simulink model "MiniDroneLogicalArchitecture_Initial"  (R2022a)
settings: Solver=VariableStepAuto  StartTime=0.0  StopTime=10.0  RelTol=1e-3
settings Model: DataDictionary=MiniDroneArchData.sldd  Creator=tshifera  LastModifiedBy=31630

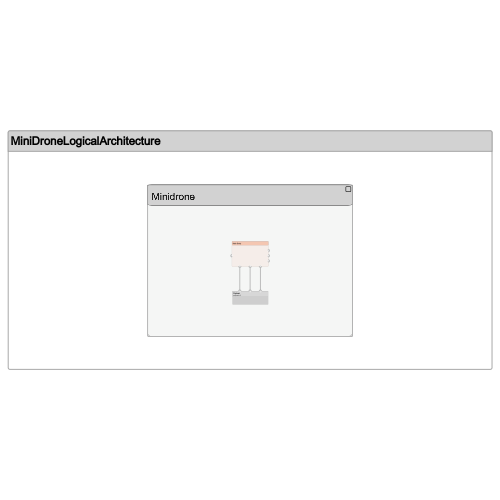
[thumbnail: Simulink's stored preview of the top-level diagram]
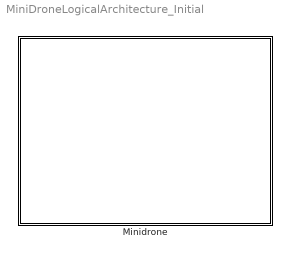
== system MiniDroneLogicalArchitecture_Initial ==
  Minidrone : Subsystem
      settings: PortSchema="{\"entries\":[{\"content\":{\"headerSize\":26,\"margin\":15,\"minimumSpacing\":25,\"sides\":[{\"content\":{\"connectorIds\":[]},\"type\":\"ConnectorPlacement.EquallySpacedRectSide\",\"uuid\":\"58971a95-43ec-4e42-90cb-f52848a43a78\"},{\"content\":{\"connectorIds\":[],\"side\":\"RIGHT\"},\"type\":\"ConnectorPlacement.EquallySpacedRectSide\",\"uuid\":\"43bd139b-3ebd-443e-9d04-2758c166e5e5\"},{\"content\":{\"connectorIds\":[],\"side\":\"TOP\"},\"type\":\"ConnectorPlacement.EquallySpacedRectSide\",\"uuid\":\"9440dd5a-d47a-4e7e-9dec-7137884490cd\"}]},\"type\":\"ConnectorPlacement.EquallySpacedConnector\",\"uuid\":\"fbcd83c6-9a27-4688-9f1d-1a4d28d86620\"}],\"packageUris\":[\"http://schema.mathworks.com/mf0/Connector/R2020b\"],\"version\":\"1.0\"}"

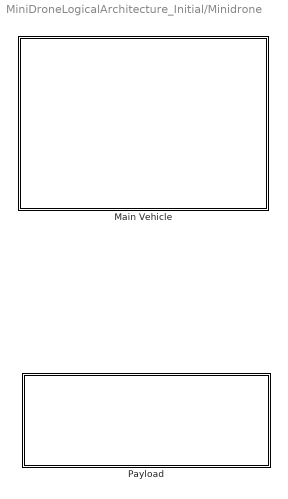
== system MiniDroneLogicalArchitecture_Initial/Minidrone ==
  Main Vehicle : Subsystem
      settings: PortSchema="{\"entries\":[{\"content\":{\"headerSize\":26,\"margin\":15,\"minimumSpacing\":25,\"sides\":[{\"content\":{\"connectorIds\":[]},\"type\":\"ConnectorPlacement.EquallySpacedRectSide\",\"uuid\":\"58971a95-43ec-4e42-90cb-f52848a43a78\"},{\"content\":{\"connectorIds\":[],\"side\":\"RIGHT\"},\"type\":\"ConnectorPlacement.EquallySpacedRectSide\",\"uuid\":\"43bd139b-3ebd-443e-9d04-2758c166e5e5\"},{\"content\":{\"connectorIds\":[],\"side\":\"TOP\"},\"type\":\"ConnectorPlacement.EquallySpacedRectSide\",\"uuid\":\"9440dd5a-d47a-4e7e-9dec-7137884490cd\"},{\"content\":{\"connectorIds\":[],\"side\":\"BOTTOM\"},\"type\":\"ConnectorPlacement.EquallySpacedRectSide\",\"uuid\":\"027f250f-1c99-4780-b31a-0472dacd58c4\"}]},\"type\":\"ConnectorPlacement.EquallySpacedConnector\",\"uuid\":\"fbcd83c6-9a27-4688-9f1d-1a4d28d86620\"}],\"packageUris\":[\"http://schema.mathworks.com/mf0/Connector/R2020b\"],\"version\":\"1.0\"}"
  Payload : Subsystem  Variant=on
      settings: PortSchema="{\"entries\":[{\"content\":{\"headerSize\":38,\"margin\":15,\"minimumSpacing\":25,\"sides\":[{\"content\":{\"connectorIds\":[]},\"type\":\"ConnectorPlacement.EquallySpacedRectSide\",\"uuid\":\"bb20ca61-cc69-46ba-bbf8-c616735728e4\"},{\"content\":{\"connectorIds\":[],\"side\":\"RIGHT\"},\"type\":\"ConnectorPlacement.EquallySpacedRectSide\",\"uuid\":\"ae599026-5f79-458c-a34f-615f09cd605e\"},{\"content\":{\"connectorIds\":[],\"side\":\"TOP\"},\"type\":\"ConnectorPlacement.EquallySpacedRectSide\",\"uuid\":\"37784589-cb93-414b-b17d-4791bb265658\"}]},\"type\":\"ConnectorPlacement.EquallySpacedConnector\",\"uuid\":\"a9e16083-13fe-49b9-9fa3-3eed0fc58f12\"}],\"packageUris\":[\"http://schema.mathworks.com/mf0/Connector/R2020b\"],\"version\":\"1.0\"}"

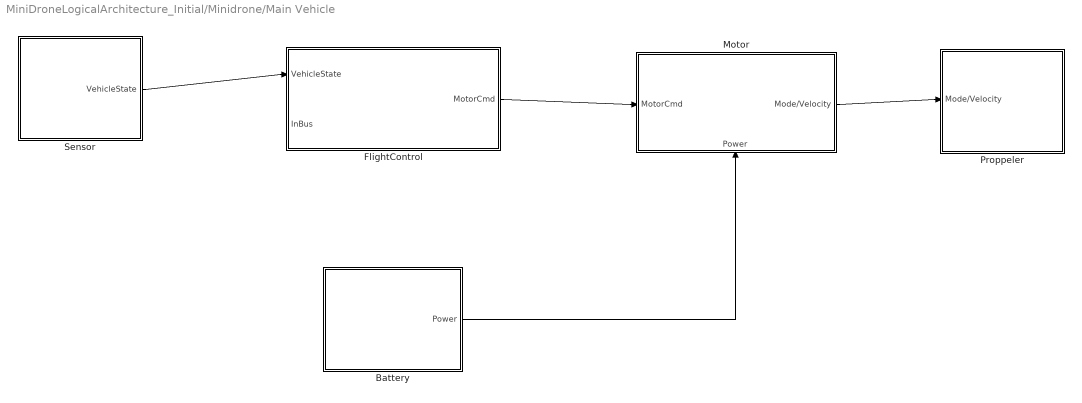
== system MiniDroneLogicalArchitecture_Initial/Minidrone/Main Vehicle ==
  Battery : Subsystem
      settings: PortSchema="{\"entries\":[{\"content\":{\"headerSize\":26,\"margin\":15,\"minimumSpacing\":25,\"sides\":[{\"content\":{\"connectorIds\":[]},\"type\":\"ConnectorPlacement.EquallySpacedRectSide\",\"uuid\":\"0bc5e52b-da78-4400-aa5e-9dddd6e99de1\"},{\"content\":{\"connectorIds\":[\"Out1\"],\"side\":\"RIGHT\"},\"type\":\"ConnectorPlacement.EquallySpacedRectSide\",\"uuid\":\"07f8a464-8fcf-4142-a2f1-5b89308ee41c\"},{\"content\":{\"connectorIds\":[],\"side\":\"TOP\"},\"type\":\"ConnectorPlacement.EquallySpacedRectSide\",\"uuid\":\"c21b697f-1019-46e9-b9d1-38a67279521c\"}]},\"type\":\"ConnectorPlacement.EquallySpacedConnector\",\"uuid\":\"700f190d-f37a-482f-bf2b-8de029522908\"}],\"packageUris\":[\"http://schema.mathworks.com/mf0/Connector/R2020b\"],\"version\":\"1.0\"}"
  FlightControl : Subsystem
      settings: PortSchema="{\"entries\":[{\"content\":{\"headerSize\":26,\"margin\":15,\"minimumSpacing\":25,\"sides\":[{\"content\":{\"connectorIds\":[\"In1\",\"In2\"]},\"type\":\"ConnectorPlacement.EquallySpacedRectSide\",\"uuid\":\"0bc5e52b-da78-4400-aa5e-9dddd6e99de1\"},{\"content\":{\"connectorIds\":[\"Out1\"],\"side\":\"RIGHT\"},\"type\":\"ConnectorPlacement.EquallySpacedRectSide\",\"uuid\":\"07f8a464-8fcf-4142-a2f1-5b89308ee41c\"},{\"content\":{\"connectorIds\":[],\"side\":\"TOP\"},\"type\":\"ConnectorPlacement.EquallySpacedRectSide\",\"uuid\":\"c21b697f-1019-46e9-b9d1-38a67279521c\"}]},\"type\":\"ConnectorPlacement.EquallySpacedConnector\",\"uuid\":\"700f190d-f37a-482f-bf2b-8de029522908\"}],\"packageUris\":[\"http://schema.mathworks.com/mf0/Connector/R2020b\"],\"version\":\"1.0\"}"
  Motor : Subsystem
      settings: PortSchema="{\"entries\":[{\"content\":{\"headerSize\":26,\"margin\":15,\"minimumSpacing\":25,\"sides\":[{\"content\":{\"connectorIds\":[\"In2\"]},\"type\":\"ConnectorPlacement.EquallySpacedRectSide\",\"uuid\":\"0bc5e52b-da78-4400-aa5e-9dddd6e99de1\"},{\"content\":{\"connectorIds\":[\"Out1\"],\"side\":\"RIGHT\"},\"type\":\"ConnectorPlacement.EquallySpacedRectSide\",\"uuid\":\"07f8a464-8fcf-4142-a2f1-5b89308ee41c\"},{\"content\":{\"connectorIds\":[],\"side\":\"TOP\"},\"type\":\"ConnectorPlacement.EquallySpacedRectSide\",\"uuid\":\"c21b697f-1019-46e9-b9d1-38a67279521c\"},{\"content\":{\"connectorIds\":[\"In1\"],\"side\":\"BOTTOM\"},\"type\":\"ConnectorPlacement.EquallySpacedRectSide\",\"uuid\":\"4b7fbe60-c35a-4c75-ab75-7f6b5398da3a\"}]},\"type\":\"ConnectorPlacement.EquallySpacedConnector\",\"uuid\":\"700f190d-f37a-482f-bf2b-8de029522908\"}],\"packageUris\":[\"http://schema.mathworks.com/mf0/Connector/R2020b\"],\"version\":\"1.0\"}"
  Proppeler : Subsystem
      settings: PortSchema="{\"entries\":[{\"content\":{\"headerSize\":26,\"margin\":15,\"minimumSpacing\":25,\"sides\":[{\"content\":{\"connectorIds\":[\"In1\"]},\"type\":\"ConnectorPlacement.EquallySpacedRectSide\",\"uuid\":\"0bc5e52b-da78-4400-aa5e-9dddd6e99de1\"},{\"content\":{\"connectorIds\":[],\"side\":\"RIGHT\"},\"type\":\"ConnectorPlacement.EquallySpacedRectSide\",\"uuid\":\"07f8a464-8fcf-4142-a2f1-5b89308ee41c\"},{\"content\":{\"connectorIds\":[],\"side\":\"TOP\"},\"type\":\"ConnectorPlacement.EquallySpacedRectSide\",\"uuid\":\"c21b697f-1019-46e9-b9d1-38a67279521c\"}]},\"type\":\"ConnectorPlacement.EquallySpacedConnector\",\"uuid\":\"700f190d-f37a-482f-bf2b-8de029522908\"}],\"packageUris\":[\"http://schema.mathworks.com/mf0/Connector/R2020b\"],\"version\":\"1.0\"}"
  Sensor : Subsystem
      settings: PortSchema="{\"entries\":[{\"content\":{\"headerSize\":26,\"margin\":15,\"minimumSpacing\":25,\"sides\":[{\"content\":{\"connectorIds\":[]},\"type\":\"ConnectorPlacement.EquallySpacedRectSide\",\"uuid\":\"0bc5e52b-da78-4400-aa5e-9dddd6e99de1\"},{\"content\":{\"connectorIds\":[\"Out1\"],\"side\":\"RIGHT\"},\"type\":\"ConnectorPlacement.EquallySpacedRectSide\",\"uuid\":\"07f8a464-8fcf-4142-a2f1-5b89308ee41c\"},{\"content\":{\"connectorIds\":[],\"side\":\"TOP\"},\"type\":\"ConnectorPlacement.EquallySpacedRectSide\",\"uuid\":\"c21b697f-1019-46e9-b9d1-38a67279521c\"}]},\"type\":\"ConnectorPlacement.EquallySpacedConnector\",\"uuid\":\"700f190d-f37a-482f-bf2b-8de029522908\"}],\"packageUris\":[\"http://schema.mathworks.com/mf0/Connector/R2020b\"],\"version\":\"1.0\"}"
  wires:
  Sensor/1(VehicleState) -> FlightControl/1(VehicleState)
  FlightControl/1(MotorCmd) -> Motor/2(MotorCmd)
  Battery/1(Power) -> Motor/1(Power)
  Motor/1(Mode/Velocity) -> Proppeler/1(Mode/Velocity)

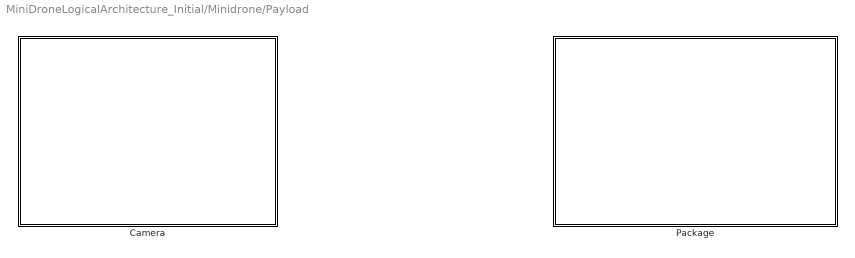
== system MiniDroneLogicalArchitecture_Initial/Minidrone/Payload ==
  Camera : Subsystem  VariantControl=payload==1
      settings: PortSchema="{\"entries\":[{\"content\":{\"headerSize\":26,\"margin\":15,\"minimumSpacing\":25,\"sides\":[{\"content\":{\"connectorIds\":[]},\"type\":\"ConnectorPlacement.EquallySpacedRectSide\",\"uuid\":\"62dbea54-6b04-428b-9082-afe16aec4c16\"},{\"content\":{\"connectorIds\":[],\"side\":\"RIGHT\"},\"type\":\"ConnectorPlacement.EquallySpacedRectSide\",\"uuid\":\"bd8afa16-d094-436c-bc9f-80902768e85a\"},{\"content\":{\"connectorIds\":[],\"side\":\"TOP\"},\"type\":\"ConnectorPlacement.EquallySpacedRectSide\",\"uuid\":\"5bc22b2d-7b46-48f6-9c81-aea78f4cffe8\"}]},\"type\":\"ConnectorPlacement.EquallySpacedConnector\",\"uuid\":\"869dc23c-b8e9-4489-a84c-3bf9ddec322d\"}],\"packageUris\":[\"http://schema.mathworks.com/mf0/Connector/R2020b\"],\"version\":\"1.0\"}"
  Package : Subsystem  VariantControl=payload==2
      settings: PortSchema="{\"entries\":[{\"content\":{\"headerSize\":26,\"margin\":15,\"minimumSpacing\":25,\"sides\":[{\"content\":{\"connectorIds\":[]},\"type\":\"ConnectorPlacement.EquallySpacedRectSide\",\"uuid\":\"62dbea54-6b04-428b-9082-afe16aec4c16\"},{\"content\":{\"connectorIds\":[],\"side\":\"RIGHT\"},\"type\":\"ConnectorPlacement.EquallySpacedRectSide\",\"uuid\":\"bd8afa16-d094-436c-bc9f-80902768e85a\"},{\"content\":{\"connectorIds\":[],\"side\":\"TOP\"},\"type\":\"ConnectorPlacement.EquallySpacedRectSide\",\"uuid\":\"5bc22b2d-7b46-48f6-9c81-aea78f4cffe8\"}]},\"type\":\"ConnectorPlacement.EquallySpacedConnector\",\"uuid\":\"869dc23c-b8e9-4489-a84c-3bf9ddec322d\"}],\"packageUris\":[\"http://schema.mathworks.com/mf0/Connector/R2020b\"],\"version\":\"1.0\"}"

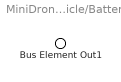
== system MiniDroneLogicalArchitecture_Initial/Minidrone/Main Vehicle/Battery ==
  Bus Element Out1 : Outport  PortName=Power

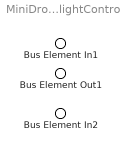
== system MiniDroneLogicalArchitecture_Initial/Minidrone/Main Vehicle/FlightControl ==
  Bus Element In1 : Inport  PortName=VehicleState
  Bus Element In2 : Inport  Port=2  PortName=InBus
  Bus Element Out1 : Outport  PortName=MotorCmd

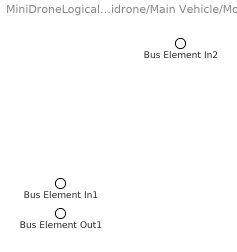
== system MiniDroneLogicalArchitecture_Initial/Minidrone/Main Vehicle/Motor ==
  Bus Element In2 : Inport  PortName=Power
  Bus Element In1 : Inport  Port=2  PortName=MotorCmd
  Bus Element Out1 : Outport  PortName=Mode/Velocity

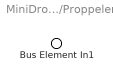
== system MiniDroneLogicalArchitecture_Initial/Minidrone/Main Vehicle/Proppeler ==
  Bus Element In1 : Inport  PortName=Mode/Velocity

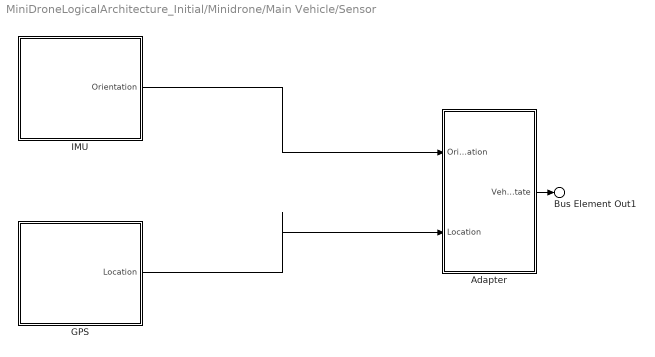
== system MiniDroneLogicalArchitecture_Initial/Minidrone/Main Vehicle/Sensor ==
  Adapter : Subsystem
      settings: PortSchema="{\"entries\":[{\"content\":{\"margin\":10,\"minimumSpacing\":15,\"sides\":[{\"content\":{\"connectorIds\":[\"In1\",\"In2\"]},\"type\":\"ConnectorPlacement.EquallySpacedRectSide\",\"uuid\":\"0bc5e52b-da78-4400-aa5e-9dddd6e99de1\"},{\"content\":{\"connectorIds\":[\"Out1\"],\"side\":\"RIGHT\"},\"type\":\"ConnectorPlacement.EquallySpacedRectSide\",\"uuid\":\"07f8a464-8fcf-4142-a2f1-5b89308ee41c\"},{\"content\":{\"connectorIds\":[],\"side\":\"TOP\"},\"type\":\"ConnectorPlacement.EquallySpacedRectSide\",\"uuid\":\"c21b697f-1019-46e9-b9d1-38a67279521c\"}]},\"type\":\"ConnectorPlacement.EquallySpacedConnector\",\"uuid\":\"700f190d-f37a-482f-bf2b-8de029522908\"}],\"packageUris\":[\"http://schema.mathworks.com/mf0/Connector/R2020b\"],\"version\":\"1.0\"}"
  GPS : Subsystem
      settings: PortSchema="{\"entries\":[{\"content\":{\"headerSize\":26,\"margin\":15,\"minimumSpacing\":25,\"sides\":[{\"content\":{\"connectorIds\":[]},\"type\":\"ConnectorPlacement.EquallySpacedRectSide\",\"uuid\":\"0bc5e52b-da78-4400-aa5e-9dddd6e99de1\"},{\"content\":{\"connectorIds\":[\"Out1\"],\"side\":\"RIGHT\"},\"type\":\"ConnectorPlacement.EquallySpacedRectSide\",\"uuid\":\"07f8a464-8fcf-4142-a2f1-5b89308ee41c\"},{\"content\":{\"connectorIds\":[],\"side\":\"TOP\"},\"type\":\"ConnectorPlacement.EquallySpacedRectSide\",\"uuid\":\"c21b697f-1019-46e9-b9d1-38a67279521c\"}]},\"type\":\"ConnectorPlacement.EquallySpacedConnector\",\"uuid\":\"700f190d-f37a-482f-bf2b-8de029522908\"}],\"packageUris\":[\"http://schema.mathworks.com/mf0/Connector/R2020b\"],\"version\":\"1.0\"}"
  IMU : Subsystem
      settings: PortSchema="{\"entries\":[{\"content\":{\"headerSize\":26,\"margin\":15,\"minimumSpacing\":25,\"sides\":[{\"content\":{\"connectorIds\":[]},\"type\":\"ConnectorPlacement.EquallySpacedRectSide\",\"uuid\":\"0bc5e52b-da78-4400-aa5e-9dddd6e99de1\"},{\"content\":{\"connectorIds\":[\"Out1\"],\"side\":\"RIGHT\"},\"type\":\"ConnectorPlacement.EquallySpacedRectSide\",\"uuid\":\"07f8a464-8fcf-4142-a2f1-5b89308ee41c\"},{\"content\":{\"connectorIds\":[],\"side\":\"TOP\"},\"type\":\"ConnectorPlacement.EquallySpacedRectSide\",\"uuid\":\"c21b697f-1019-46e9-b9d1-38a67279521c\"}]},\"type\":\"ConnectorPlacement.EquallySpacedConnector\",\"uuid\":\"700f190d-f37a-482f-bf2b-8de029522908\"}],\"packageUris\":[\"http://schema.mathworks.com/mf0/Connector/R2020b\"],\"version\":\"1.0\"}"
  Bus Element Out1 : Outport  PortName=VehicleState
  wires:
  IMU/1(Orientation) -> Adapter/1(Orientation)
  GPS/1(Location) -> Adapter/2(Location)
  Adapter/1(VehicleState) -> Bus Element Out1/1

== system MiniDroneLogicalArchitecture_Initial/Minidrone/Payload/Camera ==

== system MiniDroneLogicalArchitecture_Initial/Minidrone/Payload/Package ==

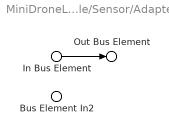
== system MiniDroneLogicalArchitecture_Initial/Minidrone/Main Vehicle/Sensor/Adapter ==
  In Bus Element : Inport  PortName=Orientation
  Bus Element In2 : Inport  Port=2  PortName=Location
  Out Bus Element : Outport  PortName=VehicleState
  wires:
  In Bus Element/1 -> Out Bus Element/1

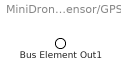
== system MiniDroneLogicalArchitecture_Initial/Minidrone/Main Vehicle/Sensor/GPS ==
  Bus Element Out1 : Outport  PortName=Location

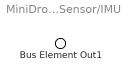
== system MiniDroneLogicalArchitecture_Initial/Minidrone/Main Vehicle/Sensor/IMU ==
  Bus Element Out1 : Outport  PortName=Orientation
